simulink model "JoystickAirshowSET1"  (R2012b)
settings: Solver=ode4  StartTime=0.0  StopTime=inf  FixedStep=sample_time  RelTol=1e-3
InitFcn:
  | sample_time=0.005;%0.004;%0.0025;%0.02;
  | sample_time_Vicon = 0.005;
  | DeltaT = 0.02;
  | g = 9.81;
  | H0 = g%0.3165;
  | Kl = 1;
  | 
  | Omega_r = 1.31;%for Horizontal reference
  | Zeta_r = 1; %for Horizontal reference
  | Omega = 1.5;%1.31;%for Horizontal Control
  | Zeta = 0.5;    %for Horizontal Control
  | 
  | Omega_h_r = 2.2; %for vertical reference
  | Zeta_h_r = 1;  %for vertical reference
  | Omega_h = 2.2;    %for vertical control
  | Zeta_h = 1;         %for vertical control
  | PI=pi;
  | 
  | Mass = 1.1;
  | Acc_Max = 4;
  | Acc_Max_h = 4;
  | 
  | Max_RP = 60;
  | 
  | % for NN
  | n = 5;
  | r = 3;
  | n2 = 5;
  | NN_ST = 0.02;
  | 
  | GAMA_V = 3;
  | gama_V_e = 0.01;
  | 
  | GAMA_W = GAMA_V;
  | gama_W_e =0.01;
  | 
  | % deadzone
  | NN_Deadzone_Z = 0;
  | 
  | % inputs nomalizaton parameters
  | NN_Z_y_min = -3;
  | NN_Z_y_max = 0.5;
  | 
  | NN_Z_v_max = 8;
  | NN_Z_v_min = -NN_Z_v_max;
  | 
  | % alpha = 0.034;
  | alpha = 1;
  | % c_f = 0.0015;
  | c_f = 0.001;
  | c_y_tilt = 1*0.5;
  | 
  | %for WK paras
  | Heightcontrol = 0.08;
  | Scale_Factor=1;
  | yoffset=0;
  | 
  | load MaoBi_Oct04_2_int.mat
  | MB_Interp.time = [];
undefined symbols (not defined in the file or in its folder): DiscIntNeverNeededParam
libraries: simulink x8, X330_Control x4, vrlib x1
(part 2 of 2)

== matlab function JoystickAirshowSET1/Planning/check if quad are too close ==
  data: Light output; Q1 input; Q2 input; Q3 input; Q5 input; BOUND output; Q5CR output; XJoy output [-3.5..3.5]; YJoy output [-3.5..3.5]; PlatformAngle data_store_memory; XJoyOut data_store_memory; YJoyOut data_store_memory; XJoyIn data_store_memory; YJoyIn data_store_memory; TangentialAngle data_store_memory; LightPWM data_store_memory
function [Light, BOUND, Q5CR,  XJoy, YJoy]   = Distance(Q1, Q2, Q3, Q5)

%  XJoyXInHalf, YJoyYInHalf, XTangentialInHalf, YTangentialInHalf,  XTangentialOutHalf, YTangentialOutHalf, XJoyXOutHalf, YJoyYOutHalf

global PlatformAngle;
global XJoyIn;
global YJoyIn;
global XJoyOut;
global YJoyOut;
global TangentialAngle;
global LightPWM;


%Distance between Joystick Quad and Formation Quad.
DQ1 = sqrt((Q5(1)-Q1(1))^2 + (Q5(2)-Q1(2))^2);
DQ2 = sqrt((Q5(1)-Q2(1))^2 + (Q5(2)-Q2(2))^2);
DQ3 = sqrt((Q5(1)-Q3(1))^2 + (Q5(2)-Q3(2))^2);


%Joystick quad current distance away from platform.


% PlatformAngle = atan2((Q5(2)-Platform(2)),(Q5(1)-Platform(1)));
PlatformAngle = atan2((Q5(1)),(Q5(2)));

%Coordinates to fly outwards while remaining 3m radius away from platform.

XJoyOut     = 3.5*sin(PlatformAngle);
YJoyOut     = 3.5*cos(PlatformAngle);

XJoyIn      = 0.4*sin(PlatformAngle);
YJoyIn      = 0.4*cos(PlatformAngle);

    
if ((DQ1<1.5)||(DQ2<1.5)||(DQ3<1.5))
    
    BOUND       = 1;
    Q5CR        = sqrt(Q5(1)^2 + Q5(2)^2);
    LightPWM    = 1250;
    Light       = LightPWM;    
      
   if(Q5CR<1.75)
       XJoy    = XJoyIn;
       YJoy    = YJoyIn;       
        
   
   elseif ((Q5CR>=1.75)&&(Q5CR<=2.45))     
       TangentialAngle = acos((sqrt(Q5(1)^2 + Q5(2)^2))/3.3);
        XJoy    = ((3.47*cos(PlatformAngle)))*sin(TangentialAngle) + ((3.47*sin(PlatformAngle)))*cos(TangentialAngle);
        YJoy    = ((3.47*cos(PlatformAngle)))*cos(TangentialAngle) - ((3.47*sin(PlatformAngle)))*sin(TangentialAngle);  
       
   
   else
       XJoy    = XJoyOut;
       YJoy    = YJoyOut;
      
   end
   
   
elseif((Q5(1)<0.4)&&(Q5(1)>-0.4)&&(Q5(2)<0.4)&&(Q5(2)>-.04)&&(Q5(3)<-1.1))
    
    BOUND       = 0;
    Q5CR        = sqrt(Q5(1)^2 + Q5(2)^2);
    LightPWM    = 1650;
    Light       = LightPWM;
    XJoy        = XJoyOut;
    YJoy        = YJoyOut;
   
elseif((Q5(1)<0.4)&&(Q5(1)>-0.4)&&(Q5(2)<0.4)&&(Q5(2)>-.04)&&(Q5(3)>-1.1))
    
    BOUND       = 0;
    Q5CR        = sqrt(Q5(1)^2 + Q5(2)^2);
    LightPWM    = 1350;
    Light       = LightPWM;
    XJoy        = XJoyOut;
    YJoy        = YJoyOut; 
    
   
elseif((Q5(1)<3.5)&&(Q5(1)>3.1)&&(Q5(2)<3)&&(Q5(2)>2.8))
    
    BOUND       = 0;
    Q5CR        = sqrt(Q5(1)^2 + Q5(2)^2);
    LightPWM    = 1650;
    Light       = LightPWM;
    XJoy        = XJoyOut;
    YJoy        = YJoyOut;
       

else
    
    BOUND       = 0;
    Q5CR        = sqrt(Q5(1)^2 + Q5(2)^2);
    Light       = LightPWM;
    
    
    if(Q5CR<2)
        XJoy    = XJoyIn;
        YJoy    = YJoyIn;
     
   
   else
        XJoy    = XJoyOut;
        YJoy    = YJoyOut;       
    
        
    end
    

end
end
